simulink model "Task_3"  (R2022b)
settings: Solver=VariableStepAuto  StartTime=0.0  StopTime=30  RelTol=1e-3
undefined symbols (not defined in the file or in its folder): A, B_2, C, C_1, D, D_1, K, L
settings Model: Creator=79211  LastModifiedBy=osini
settings DebuggingCC: UnconnectedInputMsg=warning  UnconnectedOutputMsg=warning  UnconnectedLineMsg=warning
settings ModelReferenceCC: EnableRefExpFcnMdlSchedulingChecks=on
settings RTWCC: DLArmComputeVersion=19.05

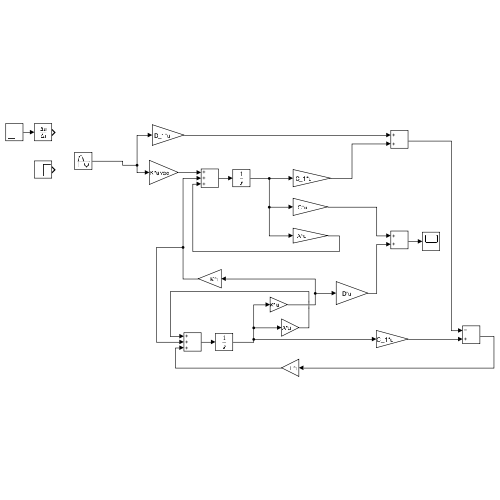
[thumbnail: Simulink's stored preview of the top-level diagram]
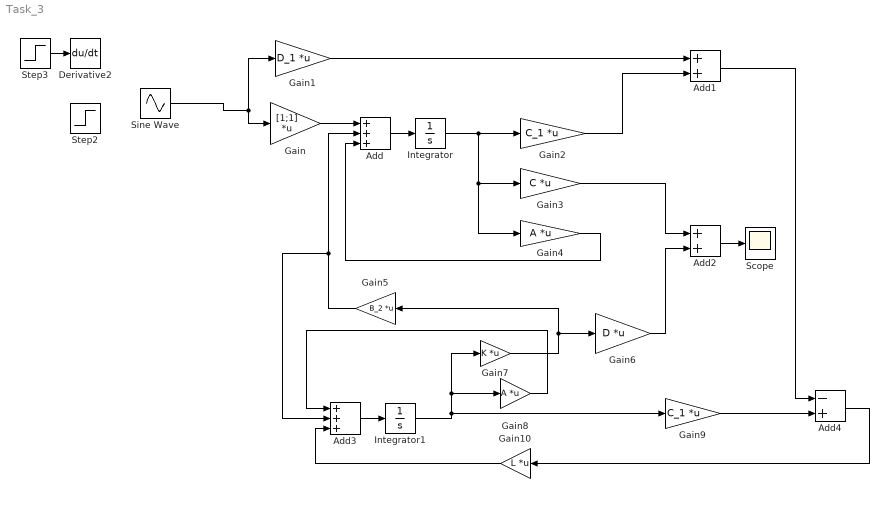
== system Task_3 ==
  Add : Sum  Inputs=+++
  Add1 : Sum
  Add2 : Sum
  Add3 : Sum  Inputs=+++
  Add4 : Sum  Inputs=-+
  Derivative2 : Derivative
  Gain : Gain  Gain=[1;1]  Multiplication=Matrix(K*u) (u vector)
  Gain1 : Gain  Gain=D_1  Multiplication=Matrix(K*u)
  Gain10 : Gain  Gain=L  Multiplication=Matrix(K*u)
  Gain2 : Gain  Gain=C_1  Multiplication=Matrix(K*u)
  Gain3 : Gain  Gain=C  Multiplication=Matrix(K*u)
  Gain4 : Gain  Gain=A  Multiplication=Matrix(K*u)
  Gain5 : Gain  Gain=B_2  Multiplication=Matrix(K*u)
  Gain6 : Gain  Gain=D  Multiplication=Matrix(K*u)
  Gain7 : Gain  Gain=K  Multiplication=Matrix(K*u)
  Gain8 : Gain  Gain=A  Multiplication=Matrix(K*u)
  Gain9 : Gain  Gain=C_1  Multiplication=Matrix(K*u)
  Integrator : Integrator
  Integrator1 : Integrator
  Scope : Scope
  Sine Wave : Sin  SampleTime=0
  Step2 : Step  SampleTime=0
  Step3 : Step  SampleTime=0
  wires:
  Gain/1 -> Add/1
  Add/1 -> Integrator/1
  Integrator/1 -> Gain4/1, Gain3/1, Gain2/1
  Gain4/1 -> Add/3
  Gain1/1 -> Add1/1
  Gain2/1 -> Add1/2
  Add1/1 -> Add4/1
  Gain3/1 -> Add2/1
  Add2/1 -> Scope/1
  Gain6/1 -> Add2/2
  Gain7/1 -> Gain5/1, Gain6/1
  Integrator1/1 -> Gain9/1, Gain7/1, Gain8/1
  Add3/1 -> Integrator1/1
  Gain8/1 -> Add3/1
  Gain9/1 -> Add4/2
  Add4/1 -> Gain10/1
  Gain5/1 -> Add3/2, Add/2
  Gain10/1 -> Add3/3
  Sine Wave/1 -> Gain/1, Gain1/1
  Step3/1 -> Derivative2/1
